simulink model "ex9"  (R2025b)
settings: Solver=ode1  StartTime=0.0  StopTime=44  MaxStep=0.05  RelTol=1e-3
libraries: simulink x13, SignalEditorBlockLib x4
settings Model: Creator=vladl  LastModifiedBy=vladl
settings ConfigComp: CovMetricSettings=dcwe

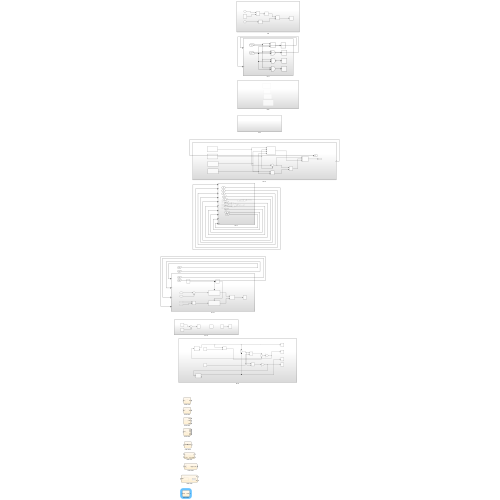
[thumbnail: Simulink's stored preview of the top-level diagram]
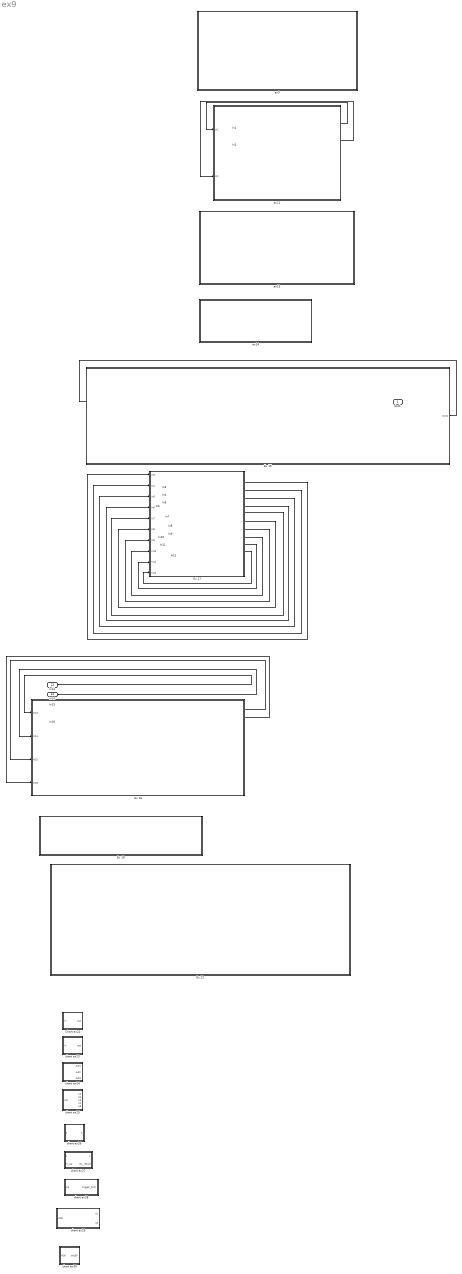
== system ex9 ==
  In1 : Inport
  In2 : Inport  Port=2
  In3 : Inport  Port=3
  In4 : Inport  Port=4
  In5 : Inport  Port=5
  In6 : Inport  Port=6
  In7 : Inport  Port=7
  In8 : Inport  Port=8
  In9 : Inport  Port=9
  In10 : Inport  Port=10
  In11 : Inport  Port=11
  In12 : Inport  Port=12
  In13 : Inport  Port=13
  In14 : Inport  Port=14
  In15 : Inport  Port=15
  In16 : Inport  Port=16
  Chart ex22 : Stateflow chart  TreatAsAtomicUnit=on
  Ex 15 : Subsystem
  Ex 16 : Subsystem
  Ex 17 : Subsystem
  Ex 18 : Subsystem
  Ex 21 : Subsystem
  chart ex23 : Stateflow chart  TreatAsAtomicUnit=on
  chart ex24 : Stateflow chart  TreatAsAtomicUnit=on
  chart ex25 : Stateflow chart  TreatAsAtomicUnit=on
  chart ex26 : Stateflow chart  TreatAsAtomicUnit=on
  chart ex27 : Stateflow chart  TreatAsAtomicUnit=on
  chart ex28 : Stateflow chart  TreatAsAtomicUnit=on
  chart ex29 : Stateflow chart  TreatAsAtomicUnit=on
  chart ex30 : Stateflow chart  TreatAsAtomicUnit=on
  ex11 : Subsystem
  ex13 : Subsystem
  ex14 : Subsystem
  ex9 : Subsystem
  Out1 : Outport
  wires:
  In1/1 -> ex11/1(In1)
  In2/1 -> ex11/2(In2)
  Ex 15/1(Out1) -> Out1/1
  In3/1 -> Ex 17/1(In3)
  In4/1 -> Ex 17/2(In4)
  In5/1 -> Ex 17/3(In5)
  In6/1 -> Ex 17/4(In6)
  In7/1 -> Ex 17/5(In7)
  In8/1 -> Ex 17/6(In8)
  In9/1 -> Ex 17/7(In9)
  In10/1 -> Ex 17/8(In10)
  In11/1 -> Ex 17/9(In11)
  In12/1 -> Ex 17/10(In12)
  In13/1 -> Ex 16/1(In13)
  In14/1 -> Ex 16/2(In14)
  In15/1 -> Ex 16/3(In15)
  In16/1 -> Ex 16/4(In16)

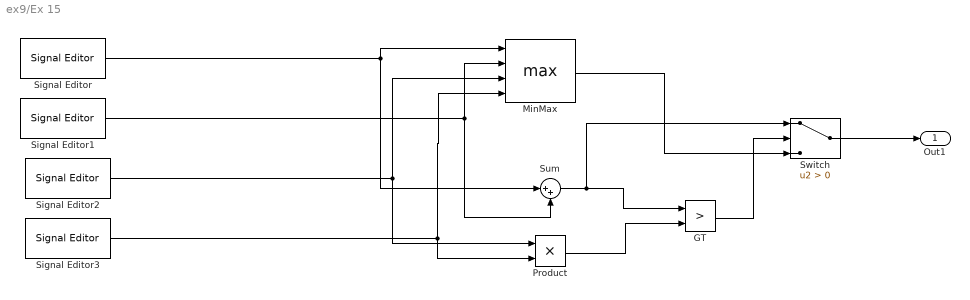
== system ex9/Ex 15 ==
  GT : RelationalOperator  Operator=>  OutDataTypeStr=boolean  RndMeth=Simplest  InputSameDT=off
  MinMax : MinMax  Function=max  Inputs=4
  Product : Product
  Signal Editor : SignalEditorBlockLib/Signal Editor  FileName=C:\Users\vladl\OneDrive\Documente\MATLAB\SIMULINK\simulink_ex15.mat  ActiveScenario=Scenario  ActiveSignal=A  IsBus=off  OutputBusObjectStr=Bus: BusObject  SampleTime=0  Interpolate=off  ZeroCross=off  OutputAfterFinalValue=Setting to zero  Unit=inherit  PreserveSignalName=on  ApplySigPropsToAllScenarios=on  ApplySigPropsToAllSignals=off  SignalPropertySource=Dialog parameters
  Signal Editor1 : SignalEditorBlockLib/Signal Editor  FileName=C:\Users\vladl\OneDrive\Documente\MATLAB\SIMULINK\ex15b.mat  ActiveScenario=Scenario  ActiveSignal=B  IsBus=off  OutputBusObjectStr=Bus: BusObject  SampleTime=0  ZeroCross=off  OutputAfterFinalValue=Setting to zero  Unit=inherit  PreserveSignalName=on  ApplySigPropsToAllScenarios=on  ApplySigPropsToAllSignals=off  SignalPropertySource=Dialog parameters
  Signal Editor2 : SignalEditorBlockLib/Signal Editor  FileName=C:\Users\vladl\OneDrive\Documente\MATLAB\SIMULINK\ex15C.mat  ActiveScenario=Scenario  ActiveSignal=C  IsBus=off  OutputBusObjectStr=Bus: BusObject  SampleTime=0  ZeroCross=off  OutputAfterFinalValue=Setting to zero  Unit=inherit  PreserveSignalName=on  ApplySigPropsToAllScenarios=on  ApplySigPropsToAllSignals=off  SignalPropertySource=Dialog parameters
  Signal Editor3 : SignalEditorBlockLib/Signal Editor  FileName=C:\Users\vladl\OneDrive\Documente\MATLAB\SIMULINK\ex15D.mat  ActiveScenario=Scenario  ActiveSignal=D  IsBus=off  OutputBusObjectStr=Bus: BusObject  SampleTime=0  ZeroCross=off  OutputAfterFinalValue=Setting to zero  Unit=inherit  PreserveSignalName=on  ApplySigPropsToAllScenarios=on  ApplySigPropsToAllSignals=off  SignalPropertySource=Dialog parameters
  Sum : Sum  Inputs=|++
  Switch : Switch  Criteria=u2 > Threshold  SaturateOnIntegerOverflow=off  InputSameDT=off
  Out1 : Outport
  wires:
  Sum/1 -> Switch/1, GT/1
  Signal Editor3/1 -> MinMax/4, Product/2
  Switch/1 -> Out1/1
  Signal Editor/1 -> MinMax/1, Sum/1
  GT/1 -> Switch/2
  Signal Editor1/1 -> Sum/2, MinMax/2
  Signal Editor2/1 -> MinMax/3, Product/1
  Product/1 -> GT/2
  MinMax/1 -> Switch/3

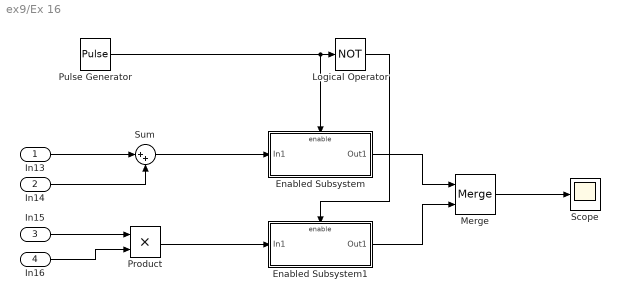
== system ex9/Ex 16 ==
  In13 : Inport
  In14 : Inport  Port=2
  In15 : Inport  Port=3
  In16 : Inport  Port=4
  Enabled Subsystem : Subsystem  TreatAsAtomicUnit=on
  Enabled Subsystem1 : Subsystem  TreatAsAtomicUnit=on
  Logical Operator : Logic  Operator=NOT  AllPortsSameDT=off  OutDataTypeStr=boolean
  Merge : Merge
  Product : Product
  Pulse Generator : DiscretePulseGenerator  PulseType=Time based  Period=10  PulseWidth=50
  Scope : Scope
      settings: DataLoggingVariableName=ScopeData21
  Sum : Sum  Inputs=|++
  wires:
  In16/1 -> Product/2
  Logical Operator/1 -> Enabled Subsystem1/Enable
  Enabled Subsystem/1(Out1) -> Merge/1
  Pulse Generator/1 -> Logical Operator/1, Enabled Subsystem/Enable
  Enabled Subsystem1/1(Out1) -> Merge/2
  Sum/1 -> Enabled Subsystem/1(In1)
  In14/1 -> Sum/2
  Product/1 -> Enabled Subsystem1/1(In1)
  In15/1 -> Product/1
  In13/1 -> Sum/1
  Merge/1 -> Scope/1

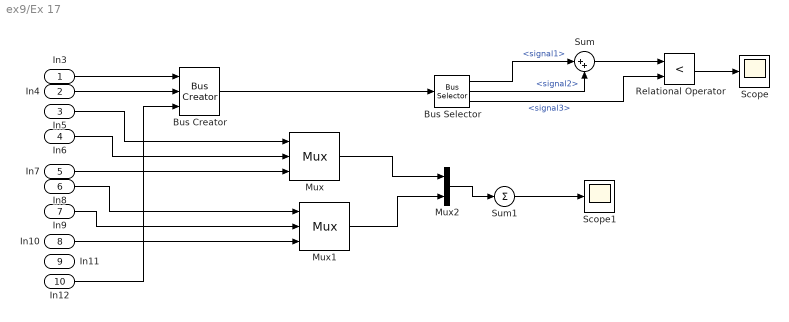
== system ex9/Ex 17 ==
  In3 : Inport
  In4 : Inport  Port=2
  In5 : Inport  Port=3
  In6 : Inport  Port=4
  In7 : Inport  Port=5
  In8 : Inport  Port=6
  In9 : Inport  Port=7
  In10 : Inport  Port=8
  In11 : Inport  Port=9
  In12 : Inport  Port=10
  Bus Creator : BusCreator  Inputs=3
  Bus Selector : BusSelector  OutputSignals=signal1,signal2,signal3
  Mux : Mux  Inputs=3
  Mux1 : Mux  Inputs=3
  Mux2 : Mux  Inputs=2
  Relational Operator : RelationalOperator  Operator=<  OutDataTypeStr=boolean  RndMeth=Simplest  InputSameDT=off
  Scope : Scope
      settings: DataLoggingVariableName=ScopeData19
  Scope1 : Scope
      settings: DataLoggingVariableName=ScopeData20
  Sum : Sum  Inputs=|++
  Sum1 : Sum  Inputs=+
  wires:
  In4/1 -> Bus Creator/2
  In3/1 -> Bus Creator/1
  In12/1 -> Bus Creator/3
  Bus Creator/1 -> Bus Selector/1
  Bus Selector/1 -> Sum/1  "<signal1>"
  Bus Selector/2 -> Sum/2  "<signal2>"
  Sum/1 -> Relational Operator/1
  Bus Selector/3 -> Relational Operator/2  "<signal3>"
  Relational Operator/1 -> Scope/1
  In5/1 -> Mux/1
  In6/1 -> Mux/2
  In7/1 -> Mux/3
  In8/1 -> Mux1/1
  In9/1 -> Mux1/2
  In10/1 -> Mux1/3
  Mux/1 -> Mux2/1
  Mux1/1 -> Mux2/2
  Mux2/1 -> Sum1/1
  Sum1/1 -> Scope1/1

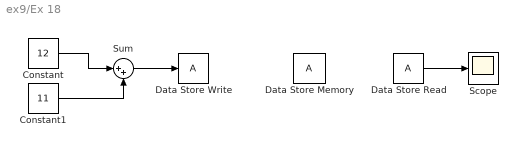
== system ex9/Ex 18 ==
  Constant : Constant  Value=12
  Constant1 : Constant  Value=11
  Data Store Memory : DataStoreMemory  WriteAfterWriteMsg=warning  ShowAdditionalParam=off
  Data Store Read : DataStoreRead  IndexOptions=Index vector (dialog)  Indices=1  OutputSizes=1
  Data Store Write : DataStoreWrite  IndexOptions=Index vector (dialog)  Indices=1  OutputSizes=1
  Scope : Scope
      settings: ActiveDisplayYMinimum=16.919333602665262  ActiveDisplayYMaximum=29.197598673480446  DataLoggingVariableName=ScopeData22
  Sum : Sum  Inputs=|++
  wires:
  Data Store Read/1 -> Scope/1
  Constant/1 -> Sum/1
  Constant1/1 -> Sum/2
  Sum/1 -> Data Store Write/1

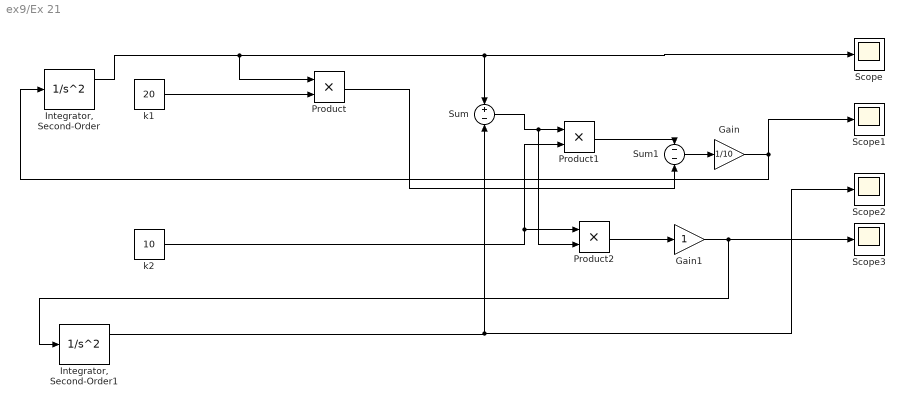
== system ex9/Ex 21 ==
  Gain : Gain  Gain=1/10
  Gain1 : Gain
  "Integrator, Second-Order" : SecondOrderIntegrator  ICX=1
  "Integrator, Second-Order1" : SecondOrderIntegrator
  Product : Product
  Product1 : Product
  Product2 : Product
  Scope{,1..3} (4 alike) : Scope
      Scope settings: ActiveDisplayYMinimum=-1.4216757762700833  ActiveDisplayYMaximum=1.2585155049799175  DataLoggingVariableName=ScopeData23
      Scope1 settings: ActiveDisplayYMinimum=-6.3467403234429671  ActiveDisplayYMaximum=5.605522446911916  DataLoggingVariableName=ScopeData24
      Scope2 settings: ActiveDisplayYMinimum=-1  ActiveDisplayYMaximum=1  DataLoggingVariableName=ScopeData25
      Scope3 settings: ActiveDisplayYMinimum=-1  ActiveDisplayYMaximum=1  DataLoggingVariableName=ScopeData26
  Sum : Sum  Inputs=+-
  Sum1 : Sum  Inputs=--
  k1 : Constant  Value=20
  k2 : Constant  Value=10
  wires:
  Gain/1 -> Scope1/1, "Integrator, Second-Order"/1
  Product/1 -> Sum1/2
  Sum/1 -> Product2/2, Product1/1
  "Integrator, Second-Order"/1 -> Scope/1, Sum/1, Product/1
  k2/1 -> Product2/1, Product1/2
  "Integrator, Second-Order1"/1 -> Scope2/1, Sum/2
  Gain1/1 -> Scope3/1, "Integrator, Second-Order1"/1
  k1/1 -> Product/2
  Product2/1 -> Gain1/1
  Product1/1 -> Sum1/1
  Sum1/1 -> Gain/1

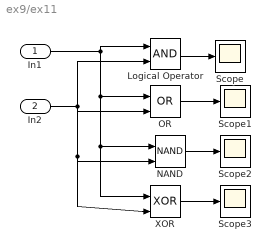
== system ex9/ex11 ==
  In1 : Inport
  In2 : Inport  Port=2
  Logical Operator : Logic  AllPortsSameDT=off  OutDataTypeStr=boolean
  NAND : Logic  Operator=NAND  IconShape=distinctive  AllPortsSameDT=off  OutDataTypeStr=boolean
  OR : Logic  Operator=OR  IconShape=distinctive  AllPortsSameDT=off  OutDataTypeStr=boolean
  Scope{,1..3} (4 alike) : Scope
      Scope settings: DataLoggingVariableName=ScopeData2
      Scope1 settings: DataLoggingVariableName=ScopeData3
      Scope2 settings: DataLoggingVariableName=ScopeData4
      Scope3 settings: DataLoggingVariableName=ScopeData5
  XOR : Logic  Operator=XOR  IconShape=distinctive  AllPortsSameDT=off  OutDataTypeStr=boolean
  wires:
  OR/1 -> Scope1/1
  In1/1 -> Logical Operator/1, XOR/1, NAND/1, OR/1
  In2/1 -> XOR/2, NAND/2, OR/2, Logical Operator/2
  NAND/1 -> Scope2/1
  Logical Operator/1 -> Scope/1
  XOR/1 -> Scope3/1

== system ex9/ex13 ==
  pule generator falling : Subsystem
  pulse generator rising : Subsystem
  signal falling : Subsystem
  signal rising : Subsystem

== system ex9/ex14 ==
  AND : Subsystem
  SET : Subsystem
  UNSET : Subsystem

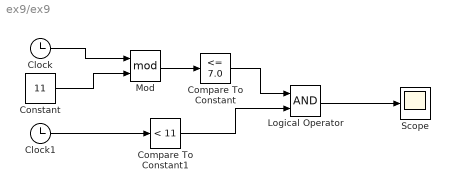
== system ex9/ex9 ==
  Clock : Clock
  Clock1 : Clock
  Compare To Constant : simulink/Logic and Bit Operations/Compare To Constant  relop=<=  const=7.0  OutDataTypeStr=boolean
  Compare To Constant1 : simulink/Logic and Bit Operations/Compare To Constant  relop=<  const=11  OutDataTypeStr=boolean
  Constant : Constant  Value=11
  Logical Operator : Logic  AllPortsSameDT=off  OutDataTypeStr=boolean
  Mod : Math  Operator=mod
  Scope : Scope
      settings: ActiveDisplayYMinimum=-2.4345295352719911  ActiveDisplayYMaximum=6.8054556493916438
  wires:
  Mod/1 -> Compare To Constant/1
  Compare To Constant1/1 -> Logical Operator/2
  Logical Operator/1 -> Scope/1
  Clock1/1 -> Compare To Constant1/1
  Constant/1 -> Mod/2
  Clock/1 -> Mod/1
  Compare To Constant/1 -> Logical Operator/1

== system ex9/Ex 16/Enabled Subsystem ==
  In1 : Inport
  Enable : EnablePort
  Out1 : Outport
  wires:
  In1/1 -> Out1/1

== system ex9/Ex 16/Enabled Subsystem1 ==
  In1 : Inport
  Enable : EnablePort
  Out1 : Outport
  wires:
  In1/1 -> Out1/1

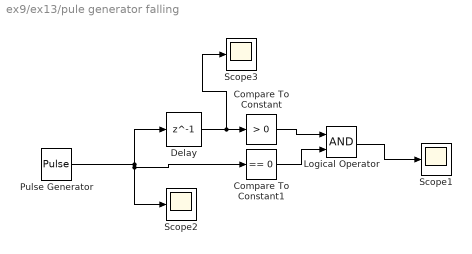
== system ex9/ex13/pule generator falling ==
  Compare To Constant : simulink/Logic and Bit Operations/Compare To Constant  relop=>  const=0  OutDataTypeStr=boolean
  Compare To Constant1 : simulink/Logic and Bit Operations/Compare To Constant  relop===  const=0  OutDataTypeStr=boolean
  Delay : Delay  DelayLength=1  InitialCondition=0
  Logical Operator : Logic  AllPortsSameDT=off  OutDataTypeStr=boolean
  Pulse Generator : DiscretePulseGenerator  PulseType=Time based  Period=10  PulseWidth=5
  Scope1 : Scope
      settings: ActiveDisplayYMinimum=-35.546525858554645  ActiveDisplayYMaximum=35.56692790033258  DataLoggingVariableName=ScopeData12
  Scope2 : Scope
      settings: ActiveDisplayYMinimum=-2.22300829387683  ActiveDisplayYMaximum=2.0528401014139552  DataLoggingVariableName=ScopeData13
  Scope3 : Scope
      settings: ActiveDisplayYMinimum=-19.662147264205881  ActiveDisplayYMaximum=18.050835582258866  DataLoggingVariableName=ScopeData14
  wires:
  Delay/1 -> Scope3/1, Compare To Constant/1
  Compare To Constant/1 -> Logical Operator/1
  Compare To Constant1/1 -> Logical Operator/2
  Pulse Generator/1 -> Compare To Constant1/1, Scope2/1, Delay/1
  Logical Operator/1 -> Scope1/1

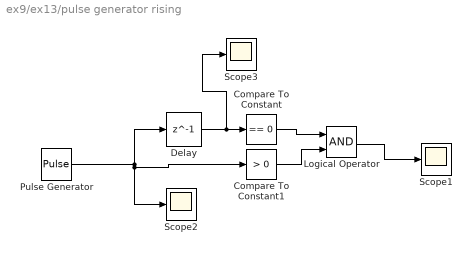
== system ex9/ex13/pulse generator rising ==
  Compare To Constant : simulink/Logic and Bit Operations/Compare To Constant  relop===  const=0  OutDataTypeStr=boolean
  Compare To Constant1 : simulink/Logic and Bit Operations/Compare To Constant  relop=>  const=0  OutDataTypeStr=boolean
  Delay : Delay  DelayLength=1  InitialCondition=0
  Logical Operator : Logic  AllPortsSameDT=off  OutDataTypeStr=boolean
  Pulse Generator : DiscretePulseGenerator  PulseType=Time based  Period=10  PulseWidth=5
  Scope1 : Scope
      settings: ActiveDisplayYMinimum=-33.814439002357474  ActiveDisplayYMaximum=37.299014756529758  DataLoggingVariableName=ScopeData11
  Scope2 : Scope
      settings: ActiveDisplayYMinimum=-2.075131769405389  ActiveDisplayYMaximum=1.4426192872352361  DataLoggingVariableName=ScopeData15
  Scope3 : Scope
      settings: ActiveDisplayYMinimum=-19.662147264205881  ActiveDisplayYMaximum=18.050835582258866  DataLoggingVariableName=ScopeData16
  wires:
  Logical Operator/1 -> Scope1/1
  Pulse Generator/1 -> Compare To Constant1/1, Scope2/1, Delay/1
  Compare To Constant/1 -> Logical Operator/1
  Delay/1 -> Scope3/1, Compare To Constant/1
  Compare To Constant1/1 -> Logical Operator/2

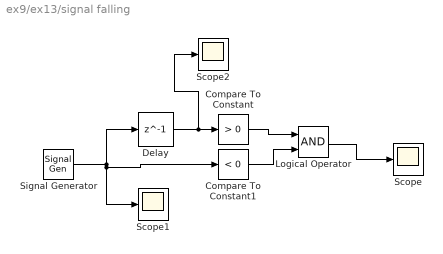
== system ex9/ex13/signal falling ==
  Compare To Constant : simulink/Logic and Bit Operations/Compare To Constant  relop=>  const=0  OutDataTypeStr=boolean
  Compare To Constant1 : simulink/Logic and Bit Operations/Compare To Constant  relop=<  const=0  OutDataTypeStr=boolean
  Delay : Delay  DelayLength=1  InitialCondition=0
  Logical Operator : Logic  AllPortsSameDT=off  OutDataTypeStr=boolean
  Scope : Scope
      settings: ActiveDisplayYMinimum=-31.838151060053441  ActiveDisplayYMaximum=29.592324058302864  DataLoggingVariableName=ScopeData8
  Scope1 : Scope
      settings: ActiveDisplayYMinimum=-2.22300829387683  ActiveDisplayYMaximum=2.0528401014139552  DataLoggingVariableName=ScopeData9
  Scope2 : Scope
      settings: ActiveDisplayYMinimum=-19.662147264205881  ActiveDisplayYMaximum=18.050835582258866  DataLoggingVariableName=ScopeData10
  Signal Generator : SignalGenerator  WaveForm=square  Units=rad/sec
  wires:
  Signal Generator/1 -> Compare To Constant1/1, Scope1/1, Delay/1
  Compare To Constant1/1 -> Logical Operator/2
  Compare To Constant/1 -> Logical Operator/1
  Delay/1 -> Scope2/1, Compare To Constant/1
  Logical Operator/1 -> Scope/1

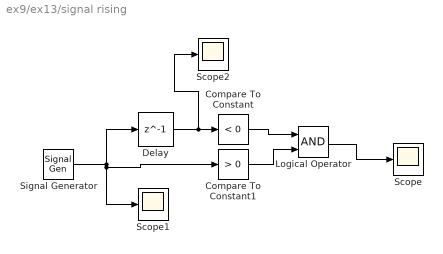
== system ex9/ex13/signal rising ==
  Compare To Constant : simulink/Logic and Bit Operations/Compare To Constant  relop=<  const=0  OutDataTypeStr=boolean
  Compare To Constant1 : simulink/Logic and Bit Operations/Compare To Constant  relop=>  const=0  OutDataTypeStr=boolean
  Delay : Delay  DelayLength=1  InitialCondition=0
  Logical Operator : Logic  AllPortsSameDT=off  OutDataTypeStr=boolean
  Scope : Scope
      settings: ActiveDisplayYMinimum=-34.682488429382254  ActiveDisplayYMaximum=39.986638017449351
  Scope1 : Scope
      settings: ActiveDisplayYMinimum=-2.22300829387683  ActiveDisplayYMaximum=2.0528401014139552  DataLoggingVariableName=ScopeData6
  Scope2 : Scope
      settings: ActiveDisplayYMinimum=-19.662147264205881  ActiveDisplayYMaximum=18.050835582258866  DataLoggingVariableName=ScopeData7
  Signal Generator : SignalGenerator  WaveForm=square  Units=rad/sec
  wires:
  Delay/1 -> Scope2/1, Compare To Constant/1
  Logical Operator/1 -> Scope/1
  Compare To Constant1/1 -> Logical Operator/2
  Compare To Constant/1 -> Logical Operator/1
  Signal Generator/1 -> Compare To Constant1/1, Scope1/1, Delay/1

== system ex9/ex14/AND ==
  Bitwise Operator : simulink/Logic and Bit Operations/Bitwise Operator  logicop=AND  UseBitMask=on  BitMask=bin2dec('00010000')  BitMaskRealWorld=Stored Integer
      settings: LibrarySourceBlock=|
      | hdlsllib/Logic and Bit
      | Operations/Bitwise
      | Operator
  Constant : Constant  Value=135  OutDataTypeStr=uint16
  Scope : Scope
      settings: ActiveDisplayYMinimum=-1  ActiveDisplayYMaximum=1  DataLoggingVariableName=ScopeData17
  wires:
  Bitwise Operator/1 -> Scope/1
  Constant/1 -> Bitwise Operator/1

== system ex9/ex14/SET ==
  Bitwise Operator1 : simulink/Logic and Bit Operations/Bitwise Operator  logicop=OR  UseBitMask=on  BitMask=bin2dec('00010000')  BitMaskRealWorld=Stored Integer
      settings: LibrarySourceBlock=|
      | hdlsllib/Logic and Bit
      | Operations/Bitwise
      | Operator
  Constant1 : Constant  Value=135  OutDataTypeStr=uint16
  Scope1 : Scope
      settings: ActiveDisplayYMinimum=-1  ActiveDisplayYMaximum=1  DataLoggingVariableName=ScopeData18
  wires:
  Constant1/1 -> Bitwise Operator1/1
  Bitwise Operator1/1 -> Scope1/1

== system ex9/ex14/UNSET ==
  Bitwise Operator1 : simulink/Logic and Bit Operations/Bitwise Operator  logicop=OR  UseBitMask=on  BitMask=bin2dec('00100000')  BitMaskRealWorld=Stored Integer
      settings: LibrarySourceBlock=|
      | hdlsllib/Logic and Bit
      | Operations/Bitwise
      | Operator
  Constant1 : Constant  Value=225  OutDataTypeStr=uint16
  Scope1 : Scope
      settings: ActiveDisplayYMinimum=-1  ActiveDisplayYMaximum=1  DataLoggingVariableName=ScopeData18
  wires:
  Constant1/1 -> Bitwise Operator1/1
  Bitwise Operator1/1 -> Scope1/1

== stateflow chart ex9/chart ex27 ==
  state y = multiplyByTen(u) [function]
    (default) -> (junction 2) : {y = u * 10;}
  state Active
    du: my_result = multiplyByTen(in_val);
  (default) -> Active
  data: u function_input; y function_output; u input; y output; in_val input; my_result output

== stateflow chart ex9/chart ex28 ==
  (default) -> (junction 4) : [in3 == 15] {trigger_fcn();}
  data: in3 input
  events: trigger_fcn output FUNCTION_CALL_EVENT

== stateflow chart ex9/chart ex29 ==
  state Active
    du: [o1, o2] = vector(in28);
  (default) -> Active
  data: in28 function_input; o1 function_output; o2 function_output; in29 input size=8; o1 output size=8; o2 output size=1; i local size=1
  function [o1, o2] = vector(in28):
    | function [o1, o2] = vector(in28)
    |     o1 = zeros(1, 8); % Initialize outputs as vectors
    |     o2 = zeros(1, 8);
    |     
    |     for i = 1:8
    |         if in28(i) == 1
    |             o1(i) = 2;
    |         else
    |             o1(i) = 3;
    |         end
    |         % Invert values (1 becomes 0, 0 becomes 1)
    |         o2(i) = 1 - in28(i); 
    |     end
    | end

== stateflow chart ex9/chart ex30 ==
  (default) -> (junction 3) [order 1] : {out30 = 0;}
  (default) -> (junction 3) [order 2] : [] {out30 = 0;}
  (junction 3) -> (junction 3) [order 1] : [rising(in30)]{out30 = 1;}
  (junction 3) -> (junction 7) [order 2]
  data: in30 input size=1; out30 output size=1

== stateflow chart ex9/chart ex23 ==
  state Passive
    du: out = out;
  state Active
    en: out = out + 1;
    du: out = out + 1;
  Active -> Passive : [in ~= 1]
  (default) -> Passive : {out = 0;}
  Passive -> Active : [in == 1]
  data: in input; out output

== stateflow chart ex9/chart ex24 ==
  state Pulse_OFF
    en: out1 = 0;
  state Pulse_ON
    out1 = 1; out3 = out3 + 1;
  state Toggle
    du: out2 ~= out2;
  Pulse_OFF -> Pulse_ON : after(100, msec)
  (default) -> Pulse_ON [order 1] : {out3 = 0;}
  (default) -> Toggle [order 2] : {out2 = 0;}
  Pulse_ON -> Pulse_OFF : after(200, msec)
  data: out1 output; out2 output; out3 output

== stateflow chart ex9/Chart ex22 ==
  (junction 15) -> (junction 17) [order 1] : [in <= 0]{out = in + 2}
  (default) -> (junction 15)
  (junction 15) -> (junction 19) [order 2] : {out = in * 2}
  data: in input; out output

== stateflow chart ex9/chart ex25 ==
  state S5
  state S4
  state S3
  state S1
  state S2
  (junction 7) -> S5 [order 3] : [in2 == 5]{s5 = s5 + 1;}
  (junction 7) -> S4 [order 2] : [in2 == 4]{s4 = s4 +1;}
  (default) -> S1 : {s1=0; s2=0; s3=0; s4=0; s5=0;}
  S1 -> (junction 7) : [in2 ~= 1]
  (junction 7) -> S1 [order 1] : [in2 == 1]{s1 = s1 + 1;}
  (junction 7) -> S3 [order 4] : [in2 == 3]{s3 = s3 + 1;}
  (junction 7) -> S2 [order 5] : [in2 == 2]{s2 = s2  + 1;}
  data: in2 input; s1 output; s2 output; s3 output; s4 output; s5 output

== stateflow chart ex9/chart ex26 ==
  state ?
  state ?
  state ?
  state ?
  state ?
  state ?
  state ?
  state ?
  state ?
  state ?
  state ?
  (junction 16) -> ? [order 3]
  (junction 16) -> ? [order 11] : [input26 == 1]{0utput26 = 10;}
  (junction 16) -> ? [order 2]
  (junction 16) -> ? [order 1]
  (junction 16) -> ? [order 4]
  (junction 16) -> ? [order 6]
  (junction 16) -> ? [order 5]
  (junction 16) -> ? [order 7]
  (junction 16) -> ? [order 10]
  (junction 16) -> ? [order 9] : [input26 ==2]{output26 =9;}
  (junction 16) -> ? [order 8]
  data: input26 input; output26 output
